simulink model "dual_mass"  (R2022a)
settings: Solver=VariableStepAuto  StartTime=0.0  StopTime=10.0  RelTol=1e-3
values from neighbouring files (symbols this model uses):
  Kflrg = 10.0    (= 10)    [parameters.m]
  Kfsm = 2.0    (= 2)    [parameters.m]
  Kvsm = 0.1    [parameters.m]
  Mlrg = 10.0    (= 10)    [parameters.m]
  Msm = 1.0    (= 1)    [parameters.m]
  U1 = 1.0    (= 1)    [parameters.m]
  U2 = 3.0    (= 3)    [parameters.m]
settings Model: Creator=Admin  LastModifiedBy=Admin

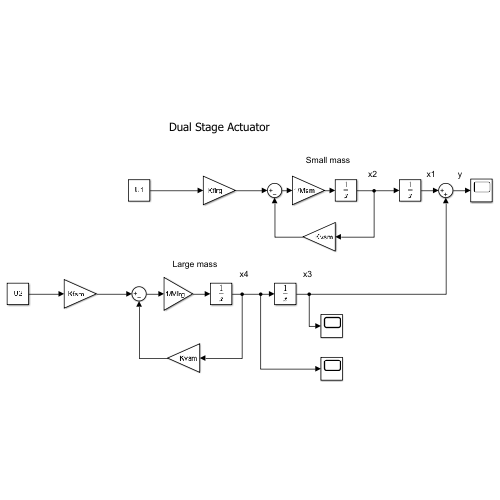
[thumbnail: Simulink's stored preview of the top-level diagram]
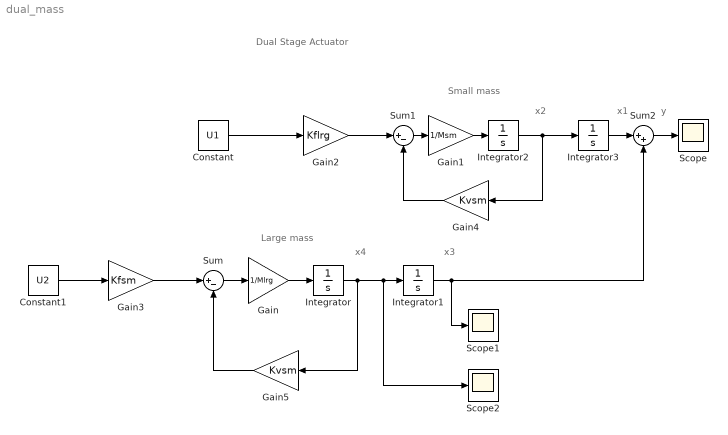
== system dual_mass ==
  note: Dual Stage Actuator
  note: y
  note: Small mass
  note: Large mass
  note: x1
  note: x2
  note: x3
  note: x4
  Constant : Constant  Value=U1
  Constant1 : Constant  Value=U2
  Gain : Gain  Gain=1/Mlrg
  Gain1 : Gain  Gain=1/Msm
  Gain2 : Gain  Gain=Kflrg
  Gain3 : Gain  Gain=Kfsm
  Gain4 : Gain  Gain=Kvsm
  Gain5 : Gain  Gain=Kvsm
  Integrator{,1..3} (4 alike) : Integrator
  Scope : Scope
  Scope1 : Scope
  Scope2 : Scope
  Sum : Sum  Inputs=|+-
  Sum1 : Sum  Inputs=|+-
  Sum2 : Sum  Inputs=|++
  wires:
  Integrator2/1 -> Gain4/1, Integrator3/1
  Integrator/1 -> Gain5/1, Scope2/1, Integrator1/1
  Gain/1 -> Integrator/1
  Sum/1 -> Gain/1
  Integrator3/1 -> Sum2/1
  Sum2/1 -> Scope/1
  Integrator1/1 -> Scope1/1, Sum2/2
  Gain3/1 -> Sum/1
  Sum1/1 -> Gain1/1
  Gain1/1 -> Integrator2/1
  Gain4/1 -> Sum1/2
  Gain5/1 -> Sum/2
  Gain2/1 -> Sum1/1
  Constant1/1 -> Gain3/1
  Constant/1 -> Gain2/1
